simulink model "engine_model2222"  (R2024b)
settings: Solver=ode4  StartTime=0.0  StopTime=10  FixedStep=1e-4  RelTol=1e-3
undefined symbols (not defined in the file or in its folder): P
libraries: simulink x7, slpidlib x1
settings Model: Creator=Administrator  LastModifiedBy=Administrator

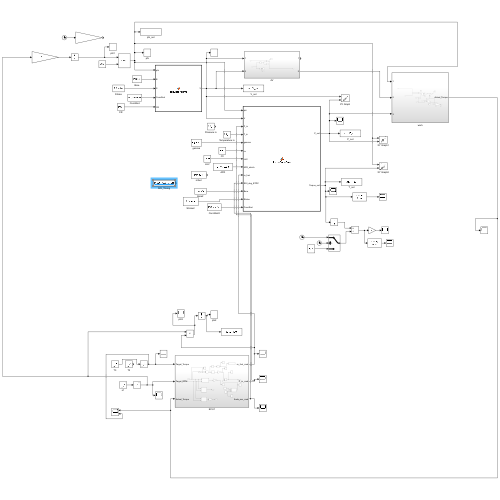
[thumbnail: Simulink's stored preview of the top-level diagram]
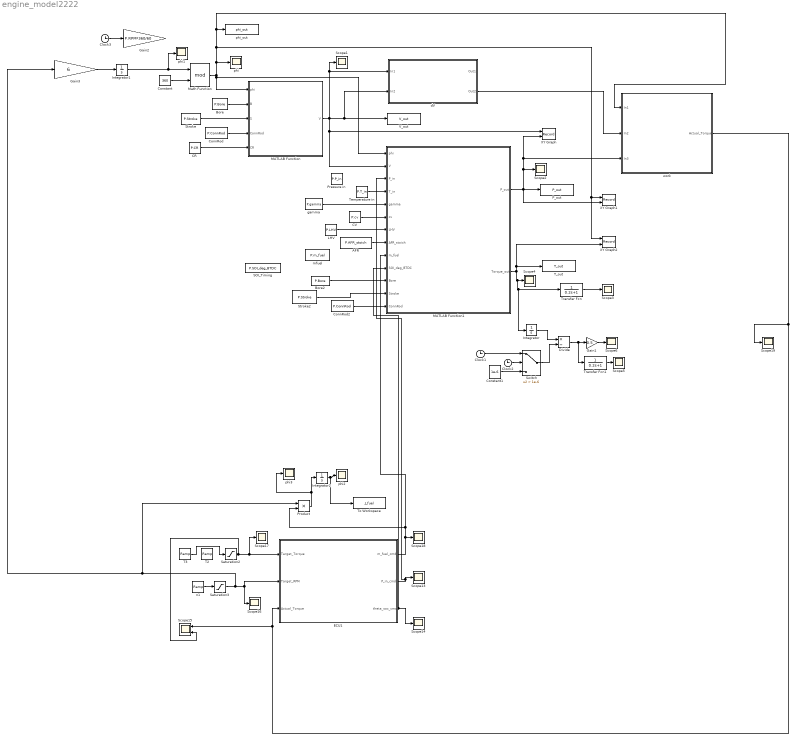
== system engine_model2222 ==
  AFR : Constant  Value=P.AFR_stoich
  Bore : Constant  Value=P.Bore
  Bore2 : Constant  Value=P.Bore
  CR : Constant  Value=P.CR
  CV : Constant  Value=P.cv
  Clock1 : Clock
  Clock2 : Clock
  Clock3 : Clock
  ConnRod : Constant  Value=P.ConnRod
  ConnRod2 : Constant  Value=P.ConnRod
  Constant : Constant  Value=360
  Constant1 : Constant  Value=1e-6
  Divide : Product  Inputs=*/
  ECU1 : Subsystem
  Gain1 : Gain  Gain=0.5
  Gain2 : Gain  Gain=P.RPM*360/60
  Gain3 : Gain  Gain=6
  Integrator : Integrator
  Integrator1 : Integrator
  Integrator2 : Integrator
  LHV : Constant  Value=P.LHV
  MATLAB Function : MATLAB Function  TreatAsAtomicUnit=on
  MATLAB Function1 : MATLAB Function  TreatAsAtomicUnit=on
  Math Function : Math  Operator=mod
  P_out : ToWorkspace  VariableName=P_out  SampleTime=-1
  Pressure in : Constant  Value=P.P_in
  Product : Product
  SOI_Timing : Constant  Value=P.SOI_deg_BTDC
  Saturation2 : Saturate  UpperLimit=450  LowerLimit=0
  Saturation3 : Saturate  UpperLimit=1800  LowerLimit=0
  Scope{1..6,13..14,16..19} (12 alike) : Scope
  Scope15 : Scope  NumInputPorts=2
  Stroke : Constant  Value=P.Stroke
  Stroke2 : Constant  Value=P.Stroke
  Switch : Switch  Criteria=u2 > Threshold  Threshold=1e-6  SaturateOnIntegerOverflow=off  InputSameDT=off
  T2 : simulink/Sources/Ramp  slope=0  start=0  InitialOutput=150  VectorParams1D=off
  T3 : simulink/Sources/Ramp  slope=41  start=0  InitialOutput=40  VectorParams1D=off
  T_out : ToWorkspace  VariableName=T_out  SampleTime=-1
  Temperature in : Constant  Value=P.T_in
  To Workspace : ToWorkspace  VariableName=J_fuel  SampleTime=-1
  Transfer Fcn : TransferFcn  Denominator=[0.2 1]
  Transfer Fcn1 : TransferFcn  Denominator=[0.2 1]
  V_out : ToWorkspace  VariableName=V_out  SampleTime=-1
  XY Graph : Record  FileSettingsInternal="{\"entries\":[{\"content\":{\"excelSettings\":{\"content\":{},\"type\":\"Streamout.ExcelSettings\"}},\"type\":\"Streamout.FileSettingStorage\",\"uuid\":\"\"}],\"packageUris\":[\"http:\\/\\/schema.mathworks.com\\/mf0\\/streamout_blocks\\/R2020a\"],\"version\":\"1.0\"}"  Layout=[1 1]  SignalsInternal="{\"entries\":[{\"content\":{\"signals\":[{\"content\":{\"blockPath\":[],\"dimensions\":[1],\"domain\":\"\",\"lineColor\":\"#a2142f\",\"lineWidth\":2,\"port\":1,\"sid\":[\"\"],\"signalID\":1,\"signalName\":\"MATLAB Function\"},\"type\":\"RecordBlkView.Signal\",\"uuid\":\"\"},{\"content\":{\"blockPath\":[],\"dimensions\":[1],\"domain\":\"\",\"lineColor\":\"#139fff\",\"lineWidth\":2,\"port\":2,\"sid\":[\"\"],\"signalID\":2,\"signalName\":\"MATLAB Function1:1\"},\"type\":\"RecordBlkView.Signal\",\"uuid\":\"\"}]},\"type\":\"RecordBlkView.InputSignals\",\"uuid\":\"\"}],\"packageUris\":[\"http:\\/\\/schema.mathworks.com\\/mf0\\/streamout_blocks\\/R2020a\"],\"version\":\"1.0\"}"  VisualizationBindings="{\"xyplotplugin\":{\"info\":[{\"series\":[],\"subplotID\":1}]}}"  CompatibilityTag=XY
  XY Graph1 : Record  FileSettingsInternal="{\"entries\":[{\"content\":{\"excelSettings\":{\"content\":{},\"type\":\"Streamout.ExcelSettings\"}},\"type\":\"Streamout.FileSettingStorage\",\"uuid\":\"\"}],\"packageUris\":[\"http:\\/\\/schema.mathworks.com\\/mf0\\/streamout_blocks\\/R2020a\"],\"version\":\"1.0\"}"  Layout=[1 1]  SignalsInternal="{\"entries\":[{\"content\":{\"signals\":[{\"content\":{\"blockPath\":[],\"dimensions\":[1,1],\"domain\":\"\",\"lineColor\":\"#fe330a\",\"lineWidth\":2,\"port\":1,\"sid\":[\"\"],\"signalID\":1,\"signalName\":\"Math\\nFunction\"},\"type\":\"RecordBlkView.Signal\",\"uuid\":\"\"},{\"content\":{\"blockPath\":[],\"dimensions\":[1],\"domain\":\"\",\"lineColor\":\"#22b573\",\"lineWidth\":2,\"port\":2,\"sid\":[\"\"],\"signalID\":2,\"signalName\":\"MATLAB Function1:1\"},\"type\":\"RecordBlkView.Signal\",\"uuid\":\"\"}]},\"type\":\"RecordBlkView.InputSignals\",\"uuid\":\"\"}],\"packageUris\":[\"http:\\/\\/schema.mathworks.com\\/mf0\\/streamout_blocks\\/R2020a\"],\"version\":\"1.0\"}"  VisualizationBindings="{\"xyplotplugin\":{\"info\":[{\"series\":[],\"subplotID\":1}]}}"  CompatibilityTag=XY
  XY Graph2 : Record  FileSettingsInternal="{\"entries\":[{\"content\":{\"excelSettings\":{\"content\":{},\"type\":\"Streamout.ExcelSettings\"}},\"type\":\"Streamout.FileSettingStorage\",\"uuid\":\"\"}],\"packageUris\":[\"http:\\/\\/schema.mathworks.com\\/mf0\\/streamout_blocks\\/R2020a\"],\"version\":\"1.0\"}"  Layout=[1 1]  SignalsInternal="{\"entries\":[{\"content\":{\"signals\":[{\"content\":{\"blockPath\":[],\"dimensions\":[1,1],\"domain\":\"\",\"lineColor\":\"#0072bd\",\"lineWidth\":2,\"port\":1,\"sid\":[\"\"],\"signalID\":1,\"signalName\":\"Math\\nFunction\"},\"type\":\"RecordBlkView.Signal\",\"uuid\":\"\"},{\"content\":{\"blockPath\":[],\"dimensions\":[1],\"domain\":\"\",\"lineColor\":\"#139fff\",\"plots\":[ 1 ],\"port\":2,\"sid\":[\"\"],\"signalID\":2,\"signalName\":\"MATLAB Function1:2\"},\"type\":\"RecordBlkView.Signal\",\"uuid\":\"\"}]},\"type\":\"RecordBlkView.InputSignals\",\"uuid\":\"\"}],\"packageUris\":[\"http:\\/\\/schema.mathworks.com\\/mf0\\/streamout_blocks\\/R2020a\"],\"version\":\"1.0\"}"  VisualizationBindings="{\"xyplotplugin\":{\"info\":[{\"series\":[{\"bindingParametersList\":[{\"parameter\":\"Y-Axis\",\"signalID\":2,\"signalName\":\"MATLAB Function1:2\"}],\"seriesID\":0}],\"subplotID\":1}]}}"  CompatibilityTag=XY
  dV : Subsystem
  gamma : Constant  Value=P.gamma
  mfuel : Constant  Value=P.m_fuel
  n1 : simulink/Sources/Ramp  slope=144  start=0  InitialOutput=360  VectorParams1D=off
  phi{,1..3} (4 alike) : Scope
  phi_out : ToWorkspace  VariableName=phi_out  SampleTime=-1
  work : Subsystem
  wires:
  Saturation3/1 -> Product/1, Gain3/1, ECU1/2(Target_RPM), Scope16/1
  Constant/1 -> Math Function/2
  Bore/1 -> MATLAB Function/2(B)
  Stroke/1 -> MATLAB Function/3(S)
  ConnRod/1 -> MATLAB Function/4(ConnRod)
  CR/1 -> MATLAB Function/5(CR)
  MATLAB Function/1(V) -> dV/1(In1), Scope1/1, dV/2(In2), V_out/1, XY Graph/1, MATLAB Function1/2(V)
  Temperature in/1 -> MATLAB Function1/4(T_in)
  gamma/1 -> MATLAB Function1/5(gamma)
  CV/1 -> MATLAB Function1/6(cv)
  LHV/1 -> MATLAB Function1/7(LHV)
  AFR/1 -> MATLAB Function1/8(AFR_stoich)
  MATLAB Function1/1(P_out) -> XY Graph/2, work/3(In3), Scope2/1, P_out/1, XY Graph1/2
  Math Function/1 -> MATLAB Function/1(phi), MATLAB Function1/1(phi), work/1(In1), phi_out/1, XY Graph2/1, XY Graph1/1, phi/1
  MATLAB Function1/2(Torque_out) -> Integrator/1, Transfer Fcn/1, Scope4/1, XY Graph2/2, T_out/1
  ConnRod2/1 -> MATLAB Function1/13(ConnRod)
  Bore2/1 -> MATLAB Function1/11(Bore)
  Stroke2/1 -> MATLAB Function1/12(Stroke)
  Transfer Fcn/1 -> Scope3/1
  Integrator/1 -> Divide/1
  Switch/1 -> Divide/2
  Divide/1 -> Transfer Fcn1/1, Gain1/1
  Clock1/1 -> Switch/1
  Clock2/1 -> Switch/2
  Constant1/1 -> Switch/3
  dV/2(Out2) -> work/2(In2)
  Transfer Fcn1/1 -> Scope5/1
  Gain1/1 -> Scope6/1
  Saturation2/1 -> Scope17/1, ECU1/1(Target_Torque), Scope15/2
  ECU1/3(theta_soc_cmd) -> Scope14/1, MATLAB Function1/10(SOI_deg_BTDC)
  n1/1 -> Saturation3/1
  work/1(Actual_Torque) -> Scope19/1, Scope15/1, ECU1/3(Actual_Torque)
  T3/1 -> Saturation2/1
  ECU1/2(P_in_cmd) -> MATLAB Function1/3(P_in), Scope13/1
  ECU1/1(m_fuel_cmd) -> Product/2, MATLAB Function1/9(m_fuel), Scope18/1
  Clock3/1 -> Gain2/1
  Gain3/1 -> Integrator1/1
  Integrator1/1 -> phi1/1, Math Function/1
  Integrator2/1 -> To Workspace/1, phi2/1
  Product/1 -> Integrator2/1, phi3/1

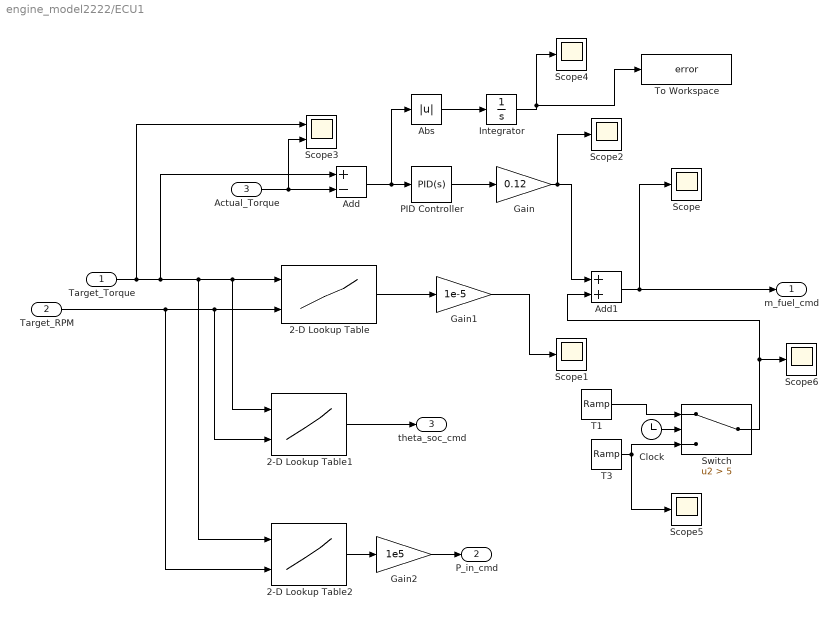
== system engine_model2222/ECU1 ==
  Target_Torque : Inport
  Target_RPM : Inport  Port=2
  Actual_Torque : Inport  Port=3
  2-D Lookup Table : Lookup_n-D  BreakpointsForDimension1=[40 150 300 450]  BreakpointsForDimension2=[360;1000;1800]  Table=[2.3 2.4 2.5;7.93 8.05 8.15;16.11 16.22 16.33;24.7 24.8 24.9]  InternalRulePriority=Speed  RndMeth=Simplest
      settings: InputPortMap=u0,u1
  2-D Lookup Table1 : Lookup_n-D  BreakpointsForDimension1=[40 150 300 450]  BreakpointsForDimension2=[360;1000;1800]  Table=[10 10 10;10 10 10;10 10 10;10 10 10]  InternalRulePriority=Speed  RndMeth=Simplest
      settings: InputPortMap=u0,u1
  2-D Lookup Table2 : Lookup_n-D  BreakpointsForDimension1=[40 150 300 450]  BreakpointsForDimension2=[360;1000;1800]  Table=[1.2 2.3 2.3;1.2 2.3 2.3;1.2 2.3 2.3;1.7 1.8 2.4]  InternalRulePriority=Speed  RndMeth=Simplest
      settings: InputPortMap=u0,u1
  Abs : Abs  SaturateOnIntegerOverflow=off
  Add : Sum  Inputs=+-
  Add1 : Sum
  Clock : Clock
  Gain : Gain  Gain=0.12
  Gain1 : Gain  Gain=1e-5
  Gain2 : Gain  Gain=1e5
  Integrator : Integrator
  PID Controller : slpidlib/PID Controller  Controller=PID  Form=Parallel  TimeDomain=Continuous-time  UseExternalTs=off  SampleTime=-1  IntegratorMethod=Forward Euler  FilterMethod=Forward Euler  ControllerParametersSource=internal  P=1  I=25  UseKiTs=on  D=0.1  UseExternalDerivativeSource=off  N=0  UseFilter=on  TunerSelectOption=Transfer Function Based (PID Tuner App)  InitialConditionSource=internal  InitialConditionForIntegrator=0  InitialConditionForFilter=0  DifferentiatorICPrevScaledInput=0  ExternalReset=none  TrackingMode=off  Kt=1  LimitOutput=on  SatLimitsSource=internal  UpperSaturationLimit=1e-4  LowerSaturationLimit=0  LinearizeAsGain=on  AntiWindupMode=none  Kb=1  LimitIntegrator=off  UpperIntegratorSaturationLimit=inf  LowerIntegratorSaturationLimit=-inf  POutMin=[]  POutMax=[]  IOutMin=[]  IOutMax=[]  DOutMin=[]  DOutMax=[]  NOutMin=[]  NOutMax=[]  SumOutMin=[]  SumOutMax=[]  SaturationOutMin=[]  SaturationOutMax=[]  PParamMin=[]  PParamMax=[]  IParamMin=[]  IParamMax=[]  DParamMin=[]  DParamMax=[]  NParamMin=[]  NParamMax=[]  KbParamMin=[]  KbParamMax=[]  KtParamMin=[]  KtParamMax=[]  KbOutMin=[]  KbOutMax=[]  KtOutMin=[]  KtOutMax=[]  IntegratorOutMin=[]  IntegratorOutMax=[]  FilterOutMin=[]  FilterOutMax=[]  SumI1OutMin=[]  SumI1OutMax=[]  SumI2OutMin=[]  SumI2OutMax=[]  SumI3OutMin=[]  SumI3OutMax=[]  SumI4OutMin=[]  SumI4OutMax=[]  SumDOutMin=[]  SumDOutMax=[]  DifferentiatorOutMin=[]  DifferentiatorOutMax=[]  FilterDiffOutCoefMin=[]  FilterDiffOutCoefMax=[]  ReciprocalOutMin=[]  ReciprocalOutMax=[]  SumDenOutMin=[]  SumDenOutMax=[]  SumNumOutMin=[]  SumNumOutMax=[]  DivideOutMin=[]  DivideOutMax=[]  UdiffTsProdOutMin=[]  UdiffTsProdOutMax=[]  NTsProdOutMin=[]  NTsProdOutMax=[]  UintegralTsProdOutMin=[]  UintegralTsProdOutMax=[]  UngainTsProdOutMin=[]  UngainTsProdOutMax=[]  ClampingZeroOutDataTypeStr=Inherit: Inherit via back propagation  ClampingZeroOutMin=[]  ClampingZeroOutMax=[]  FilterDenConstantOutDataTypeStr=Inherit: Inherit via back propagation  FilterDenConstantOutMin=[]  FilterDenConstantOutMax=[]  PCopyOutDataTypeStr=Inherit: Inherit via back propagation  PCopyOutMin=[]  PCopyOutMax=[]  NCopyOutDataTypeStr=Inherit: Inherit via back propagation  NCopyOutMin=[]  NCopyOutMax=[]  IntegratorContinuousStateAttributes=''  IntegratorStateMustResolveToSignalObject=off  IntegratorRTWStateStorageClass=Auto  FilterContinuousStateAttributes=''  FilterStateMustResolveToSignalObject=off  FilterRTWStateStorageClass=Auto  ParallelPVariant=InternalParameters  IdealPVariant=Disabled  IVariant=InternalParameters  DVariant=InternalParameters  IntegratorVariant=Continuous  SatVariant=Enabled  AWVariant=Passthrough  PCopyVariant=Disabled  TRVariant=Disabled  FdbkBlocksVariant=Forward  IdealPFdbkVariant=Disabled  SatFdbkVariant=Disabled  DerivativeFilterVariant=ContFilter  NVariant=InternalParameters  NCopyVariant=Disabled  FilterICVariant=InternalICsFilter  IntegratorICVariant=InternalICs  ExternalResetVariant=Disabled  TRSumVariant=Passthrough  SumFdbkVariant=Disabled  SumVariant=Sum_PID  TsampFilterVariant=InternalTs  TsampNgainVariant=Passthrough  TsampIntegralVariant=Disabled_SignalSpec  ExternalSaturationOutDataTypeStr=Inherit: Same as second input  DerivativeSourceVariant=ErrorSignal  PreIntVariant=InternalPreInt
  Scope{,1..2,4..6} (6 alike) : Scope
  Scope3 : Scope  NumInputPorts=2
  Switch : Switch  Criteria=u2 > Threshold  Threshold=5  SaturateOnIntegerOverflow=off  InputSameDT=off
  T1 : simulink/Sources/Ramp  slope=2.275e-5  start=0  InitialOutput=2.3e-5  VectorParams1D=off
  T3 : simulink/Sources/Ramp  slope=2.3e-5  start=0  InitialOutput=2.3e-5  VectorParams1D=off
  To Workspace : ToWorkspace  VariableName=error  SampleTime=-1
  m_fuel_cmd : Outport
  P_in_cmd : Outport  Port=2
  theta_soc_cmd : Outport  Port=3
  wires:
  Target_Torque/1 -> Scope3/1, Add/1, 2-D Lookup Table2/1, 2-D Lookup Table1/1, 2-D Lookup Table/1
  Target_RPM/1 -> 2-D Lookup Table2/2, 2-D Lookup Table1/2, 2-D Lookup Table/2
  Actual_Torque/1 -> Scope3/2, Add/2
  Add/1 -> Abs/1, PID Controller/1
  PID Controller/1 -> Gain/1
  2-D Lookup Table/1 -> Gain1/1
  Gain/1 -> Scope2/1, Add1/1
  Add1/1 -> m_fuel_cmd/1, Scope/1
  2-D Lookup Table1/1 -> theta_soc_cmd/1
  Gain1/1 -> Scope1/1
  Abs/1 -> Integrator/1
  Integrator/1 -> To Workspace/1, Scope4/1
  Gain2/1 -> P_in_cmd/1
  2-D Lookup Table2/1 -> Gain2/1
  T3/1 -> Scope5/1, Switch/3
  Switch/1 -> Scope6/1, Add1/2
  Clock/1 -> Switch/2
  T1/1 -> Switch/1

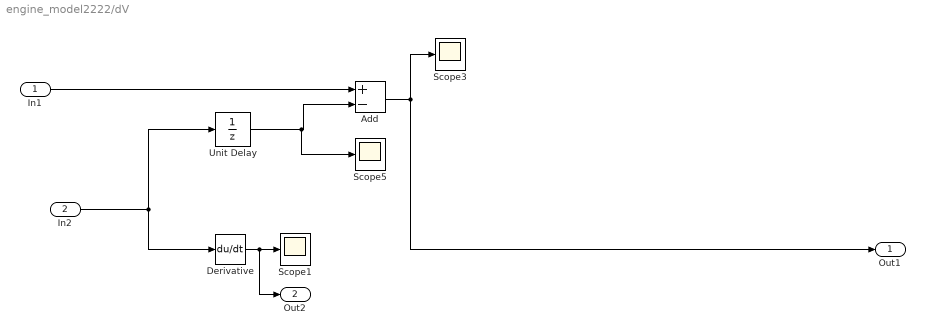
== system engine_model2222/dV ==
  In1 : Inport
  In2 : Inport  Port=2
  Add : Sum  Inputs=+-
  Derivative : Derivative
  Scope1 : Scope
  Scope3 : Scope
  Scope5 : Scope
  Unit Delay : UnitDelay  InitialCondition=2.6e-3  SampleTime=-1  HasFrameUpgradeWarning=on
  Out1 : Outport
  Out2 : Outport  Port=2
  wires:
  Unit Delay/1 -> Scope5/1, Add/2
  In2/1 -> Unit Delay/1, Derivative/1
  Add/1 -> Out1/1, Scope3/1
  In1/1 -> Add/1
  Derivative/1 -> Out2/1, Scope1/1

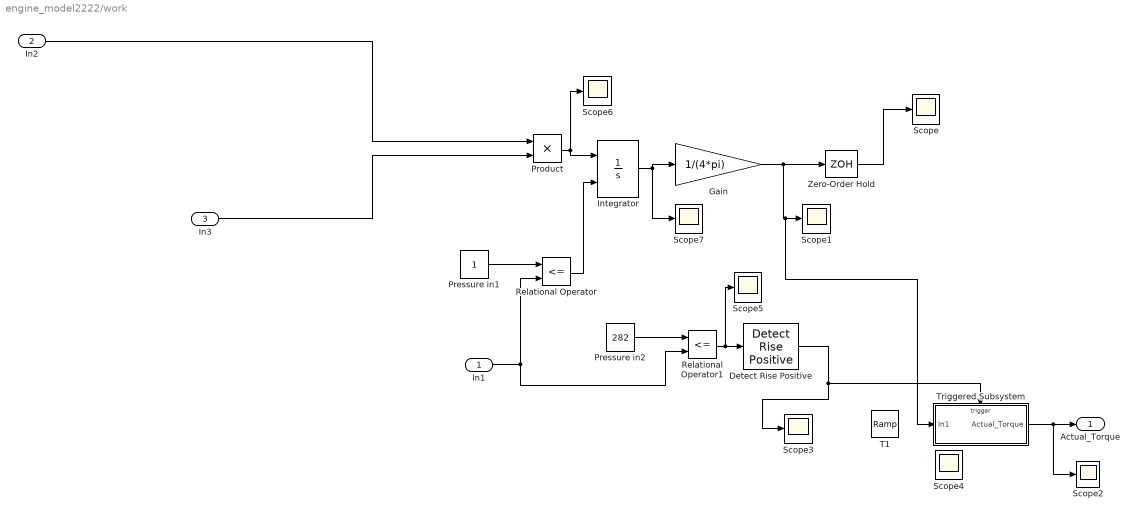
== system engine_model2222/work ==
  In1 : Inport
  In2 : Inport  Port=2
  In3 : Inport  Port=3
  Detect Rise Positive : simulink/Logic and Bit Operations/Detect Rise Positive  vinit=0  OutDataTypeStr=boolean
  Gain : Gain  Gain=1/(4*pi)
  Integrator : Integrator  ExternalReset=rising
  Pressure in1 : Constant
  Pressure in2 : Constant  Value=282
  Product : Product
  Relational Operator : RelationalOperator  Operator=<=  OutDataTypeStr=boolean  RndMeth=Simplest  InputSameDT=off
  Relational Operator1 : RelationalOperator  Operator=<=  OutDataTypeStr=boolean  RndMeth=Simplest  InputSameDT=off
  Scope{,1..7} (8 alike) : Scope
  T1 : simulink/Sources/Ramp  slope=410  start=0  InitialOutput=40  VectorParams1D=off
  Triggered Subsystem : Subsystem  TreatAsAtomicUnit=on
  Zero-Order Hold : ZeroOrderHold  SampleTime=round(60*10000/P.RPM)/10000
  Actual_Torque : Outport
  wires:
  Integrator/1 -> Gain/1, Scope7/1
  In3/1 -> Product/2
  Relational Operator/1 -> Integrator/2
  Product/1 -> Scope6/1, Integrator/1
  Pressure in1/1 -> Relational Operator/1
  In2/1 -> Product/1
  Gain/1 -> Zero-Order Hold/1, Triggered Subsystem/1(In1), Scope1/1
  Zero-Order Hold/1 -> Scope/1
  Triggered Subsystem/1(Actual_Torque) -> Actual_Torque/1, Scope2/1
  Pressure in2/1 -> Relational Operator1/1
  In1/1 -> Relational Operator/2, Relational Operator1/2
  Relational Operator1/1 -> Scope5/1, Detect Rise Positive/1
  Detect Rise Positive/1 -> Scope3/1, Triggered Subsystem/Trigger

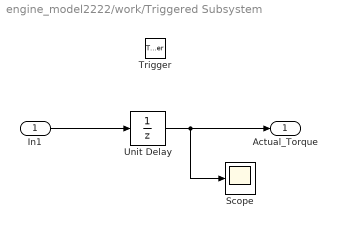
== system engine_model2222/work/Triggered Subsystem ==
  In1 : Inport
  Trigger : TriggerPort  VariantControl=(inherit)
  Scope : Scope
  Unit Delay : UnitDelay  SampleTime=-1  HasFrameUpgradeWarning=on
  Actual_Torque : Outport
  wires:
  In1/1 -> Unit Delay/1
  Unit Delay/1 -> Scope/1, Actual_Torque/1

== matlab function engine_model2222/MATLAB Function1 ==
  settings: updateMethod=DISCRETE
  data: phi input; P_out output; V input; P_in input; T_in input; gamma input; cv input; LHV input; AFR_stoich input; m_fuel input; SOI_deg_BTDC input; Bore input; Stroke input; ConnRod input; Torque_out output
function [P_out, Torque_out] = thermoCycleCore(phi, V, P_in, T_in, gamma, cv, LHV, AFR_stoich, m_fuel, SOI_deg_BTDC, Bore, Stroke, ConnRod)
% =========================================================================
% 这是热力学核心的【V7 - 包含扭矩输出版】
% 输出: 压力(P_out), 温度(T_out), 和瞬时扭矩(Torque_out)
% =========================================================================
P_out=1e5;
% persistent 变量用于在仿真步之间保存状态
persistent P_state T_state V_state process_state m_air;

% ---- 初始化 ----
if isempty(process_state) || phi < 1
process_state = 1; % 1=压缩, 2=燃烧, 3=膨胀
V_state = V;
P_state = P_in;
T_state = T_in;
m_air = (P_in * V_state) / (287 * T_state);
end

% ---- 状态机逻辑 ----
combustion_angle = 180 - SOI_deg_BTDC;

% 1. 压缩过程 (Compression)
if process_state == 1
if phi < combustion_angle
P_out = P_state * (V_state / V)^gamma;

else % 到达燃烧点，切换到状态2
% 在切换的瞬间，需要先给输出赋值，否则会报错
P_out = P_state * (V_state / V)^gamma;

process_state = 2;
end
end

% 2. 燃烧过程 (Combustion) - 这是一个瞬时过程
if process_state == 2
P_comp_end = P_state * (V_state / V)^gamma;
T_comp_end = T_state * (V_state / V)^(gamma-1);

equivalence_ratio = (m_fuel / m_air) * AFR_stoich;
if equivalence_ratio <= 1
m_fuel_burned = m_fuel;
else
m_fuel_burned = m_air / AFR_stoich;
end

Q_in = m_fuel_burned * LHV;
delta_T = Q_in / (m_air * cv);

T_out = T_comp_end + delta_T;
P_out = P_comp_end * (T_out / T_comp_end);

% 更新状态，为膨胀过程做准备
P_state = P_out;
T_state = T_out;
V_state = V;
process_state = 3; % 切换到膨胀状态
end

% 3. 膨胀过程 (Expansion)
if process_state == 3
if phi < 360
P_out = P_state * (V_state / V)^gamma;

else
P_out = P_in;

end
end

% 确保在循环的最后阶段输出的是进气压力
if phi >= 360
P_out = P_in;

end


% =========================================================================
% ### 新增：瞬时扭矩计算部分 ###
% =========================================================================
% 几何参数
a = Stroke / 2; % 曲柄半径 (m)
L = ConnRod; % 连杆长度 (m)
Ap = (pi/4) * Bore^2; % 活塞面积 (m^2)

% 将Simulink的0-360度循环角度转换为以压缩上止点(TDC)为0度的数学角度
% phi_math_rad 的范围是 -pi 到 +pi
phi_math_rad = deg2rad(phi - 180);

% 计算连杆角度 beta (rad)
% 添加一个小的epsilon (1e-8) 来防止 asin 的输入因浮点误差略大于1而报错
arg = (a/L) * sin(phi_math_rad);
if abs(arg) > 1
arg = sign(arg);
end
beta = asin(arg);

% 作用在活塞上的力 (N) (忽略曲轴箱压力)
F_piston = P_out * Ap;

% 瞬时扭矩公式 (N·m)
Torque_out = F_piston * a * sin(phi_math_rad + beta) / cos(beta);

end

== matlab function engine_model2222/MATLAB Function ==
  data: phi input; V output; B input; S input; ConnRod input; CR input
function V = calculateVolume(phi, B, S, ConnRod, CR)
% 输入:
% phi: 当前曲轴转角 (度)
% 输出:
% V: 瞬时气缸容积 (m^3)

a = S / 2; % 曲柄半径
R = ConnRod / a;

V_swept = (pi/4) * B^2 * S; % 排量
V_c = V_swept / (CR - 1); % 余隙容积

% 将0-360度的输入转换为-180到+180度，以匹配公式中TDC=0度的习惯
phi_math = phi - 180;
phi_rad = deg2rad(phi_math);

x = a * (R + 1 - cos(phi_rad) - sqrt(R^2 - sin(phi_rad)^2));
V = V_c + (pi/4) * B^2 * x;
end
